simulink model "pendeLAI"  (Simulink 6.0)
settings: Solver=ode45  StartTime=0.0  StopTime=100.0  RelTol=1e-4
values from neighbouring files (symbols this model uses):
  PMswitch = 1    [quadresp_sim.m]    (also in quadresp_sim_2.m)
  UIMswitch = 1    [quadresp_sim.m]    (also in quadresp_sim_2.m)
libraries: cstblocks x15
settings Model: Creator=rana  LastModifiedBy=Administrator  ExtModeTrigMode=oneshot  ExtModeArmWhenConnect=off  ExtModeAutoUpdateStatusClock=off
settings DataIOCC: LimitDataPoints=off
settings OptimizationCC: BlockReduction=off  BooleanDataType=off
settings DebuggingCC: SolverPrmCheckMsg=none  UnconnectedInputMsg=none  UnconnectedOutputMsg=none
settings HardwareCC: TargetUnknown=on
settings GRTTargetCC: ModelReferenceCompliant=off  MatFileLogging=off

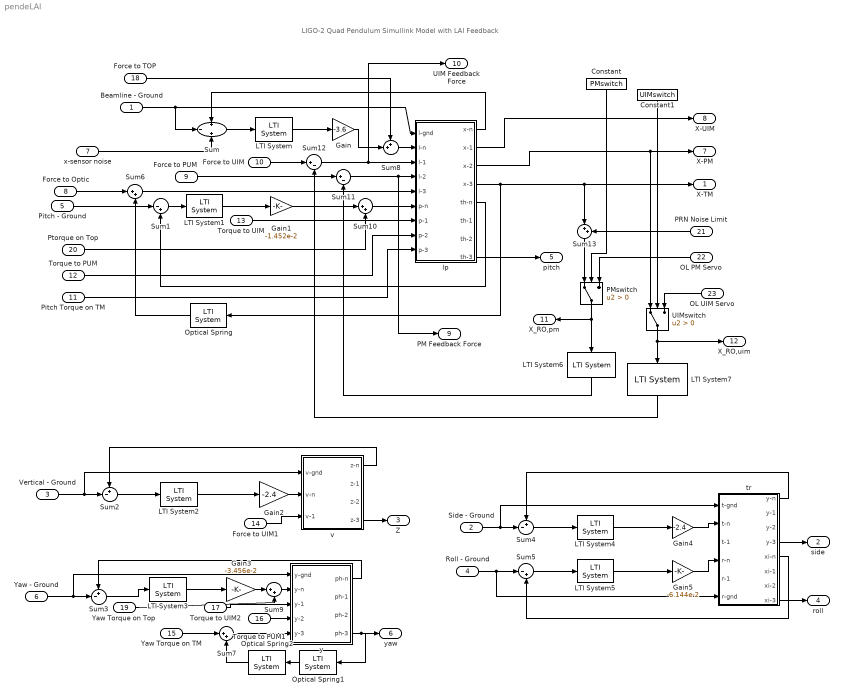
== system pendeLAI ==
  note: LIGO-2 Quad Pendulum Simullink Model
      | with LAI Feedback
  Beamline - Ground : Inport  Port=1  LatchInput=off
  Side - Ground : Inport  Port=2  LatchInput=off
  Vertical - Ground : Inport  Port=3  LatchInput=off
  Roll - Ground : Inport  Port=4  LatchInput=off
  Pitch - Ground : Inport  Port=5  LatchInput=off
  Yaw - Ground : Inport  Port=6  LatchInput=off
  x-sensor noise : Inport  Port=7  LatchInput=off
  Force to Optic : Inport  Port=8  LatchInput=off
  Force to PUM : Inport  Port=9  LatchInput=off
  Force to UIM : Inport  Port=10  LatchInput=off
  Pitch Torque on TM : Inport  Port=11  LatchInput=off
  Torque to PUM : Inport  Port=12  LatchInput=off
  Torque to UIM : Inport  Port=13  LatchInput=off
  Force to UIM1 : Inport  Port=14  LatchInput=off
  Yaw Torque on TM : Inport  Port=15  LatchInput=off
  Torque to PUM1 : Inport  Port=16  LatchInput=off
  Torque to UIM2 : Inport  Port=17  LatchInput=off
  Force to TOP : Inport  Port=18  LatchInput=off
  Yaw Torque on Top : Inport  Port=19  LatchInput=off
  Ptorque on Top : Inport  Port=20  LatchInput=off
  PRN Noise Limit : Inport  Orientation=left  Port=21  LatchInput=off
  OL PM Servo : Inport  Orientation=left  Port=22  LatchInput=off
  OL UIM Servo : Inport  Orientation=left  Port=23  LatchInput=off
  Constant : Constant  Orientation=down  Value=PMswitch
  Constant1 : Constant  Orientation=down  Value=UIMswitch
  Gain : Gain  Gain=-3.6
  Gain1 : Gain  Gain=-1.452e-2
  Gain2 : Gain  Gain=-2.4
  Gain3 : Gain  Gain=-3.456e-2
  Gain4 : Gain  Gain=-2.4
  Gain5 : Gain  Gain=-6.144e-2
  LTI System : cstblocks/LTI System  sys=ldamp  IC=0
  LTI System1 : cstblocks/LTI System  sys=pdamp  IC=0
  LTI System2 : cstblocks/LTI System  sys=vdamp  IC=0
  LTI System3 : cstblocks/LTI System  sys=ydamp  IC=0
  LTI System4 : cstblocks/LTI System  sys=tdamp  IC=0
  LTI System5 : cstblocks/LTI System  sys=rdamp  IC=0
  LTI System6 : cstblocks/LTI System  Orientation=down  sys=ServoPM  IC=[]
  LTI System7 : cstblocks/LTI System  Orientation=down  sys=ServoUIM  IC=[]
  Optical Spring : cstblocks/LTI System  Orientation=left  sys=k_ospring  IC=[]
  Optical Spring1 : cstblocks/LTI System  Orientation=left  sys=k_major  IC=[]
  Optical Spring2 : cstblocks/LTI System  Orientation=left  sys=k_minor  IC=[]
  PMswitch : Switch  Orientation=down  Criteria=u2 > Threshold
  Sum : Sum  Inputs=+|-|+  InputSameDT=on
  Sum1 : Sum  Inputs=|-+  InputSameDT=on
  Sum{6..7,9..10} (4 alike) : Sum  Inputs=|++  InputSameDT=on
  Sum11 : Sum  Inputs=|+-  InputSameDT=on
  Sum12 : Sum  Inputs=|+-  InputSameDT=on
  Sum13 : Sum  Orientation=down  Inputs=|++  InputSameDT=on
  Sum2 : Sum  Inputs=+-|  InputSameDT=on
  Sum3 : Sum  Inputs=+-|  InputSameDT=on
  Sum4 : Sum  Inputs=+-|  InputSameDT=on
  Sum5 : Sum  Inputs=|-+  InputSameDT=on
  Sum8 : Sum  Inputs=++|  InputSameDT=on
  UIMswitch : Switch  Orientation=down  Criteria=u2 > Threshold
  lp : Subsystem
  tr : Subsystem
  v : Subsystem
  y : Subsystem
  X-TM : Outport
  side : Outport  Port=2
  Z : Outport  Port=3
  roll : Outport  Port=4
  pitch : Outport  Port=5
  yaw : Outport  Port=6
  X-PM : Outport  Port=7
  X-UIM : Outport  Port=8
  PM Feedback Force : Outport  Port=9
  UIM Feedback Force : Outport  Port=10
  X_RO,pm : Outport  Orientation=left  Port=11
  X_RO,uim : Outport  Port=12
  wires:
  Gain2/1 -> v/2(v-n)
  Gain4/1 -> tr/2(t-n)
  Gain5/1 -> tr/4(r-n)
  Gain1/1 -> Sum10/1
  y/1(ph-n) -> Sum3/1
  tr/5(xi-n) -> Sum5/2
  tr/1(y-n) -> Sum4/1
  lp/5(th-n) -> Sum1/2
  lp/1(x-n) -> Sum/1
  LTI System/1 -> Gain/1
  Sum1/1 -> LTI System1/1
  Sum3/1 -> LTI System3/1
  Sum4/1 -> LTI System4/1
  Sum5/1 -> LTI System5/1
  v/1(z-n) -> Sum2/1
  Sum/1 -> LTI System/1
  Sum2/1 -> LTI System2/1
  Beamline - Ground/1 -> lp/1(l-gnd), Sum/2
  Pitch - Ground/1 -> Sum1/1
  Vertical - Ground/1 -> Sum2/2, v/1(v-gnd)
  Yaw - Ground/1 -> Sum3/2, y/1(y-gnd)
  Side - Ground/1 -> Sum4/2, tr/1(t-gnd)
  Roll - Ground/1 -> Sum5/1, tr/6(r-gnd)
  lp/4(x-3) -> Optical Spring/1, X-TM/1, Sum13/1
  tr/4(y-3) -> side/1
  v/4(z-3) -> Z/1
  tr/8(xi-3) -> roll/1
  lp/8(th-3) -> pitch/1
  y/4(ph-3) -> Optical Spring1/1, yaw/1
  LTI System1/1 -> Gain1/1
  LTI System2/1 -> Gain2/1
  LTI System3/1 -> Gain3/1
  LTI System4/1 -> Gain4/1
  LTI System5/1 -> Gain5/1
  x-sensor noise/1 -> Sum/3
  Pitch Torque on TM/1 -> lp/9(p-3)
  Torque to PUM/1 -> lp/8(p-2)
  Torque to UIM/1 -> lp/7(p-1)
  Force to Optic/1 -> Sum6/1
  Sum6/1 -> lp/5(l-3)
  Optical Spring/1 -> Sum6/2
  Force to UIM1/1 -> v/3(v-1)
  Torque to UIM2/1 -> y/3(y-1)
  Torque to PUM1/1 -> y/4(y-2)
  Yaw Torque on TM/1 -> Sum7/1
  Sum7/1 -> y/5(y-3)
  Optical Spring1/1 -> Optical Spring2/1
  Optical Spring2/1 -> Sum7/2
  Gain/1 -> Sum8/2
  Sum8/1 -> lp/2(I-n)
  Force to TOP/1 -> Sum8/1
  Gain3/1 -> Sum9/1
  Sum9/1 -> y/2(y-n)
  Yaw Torque on Top/1 -> Sum9/2
  Sum10/1 -> lp/6(p-n)
  Ptorque on Top/1 -> Sum10/2
  lp/3(x-2) -> X-PM/1, UIMswitch/1
  lp/2(x-1) -> X-UIM/1
  Sum11/1 -> lp/4(l-2), PM Feedback Force/1
  Force to PUM/1 -> Sum11/1
  LTI System6/1 -> Sum11/2
  Sum12/1 -> lp/3(l-1), UIM Feedback Force/1
  Force to UIM/1 -> Sum12/1
  LTI System7/1 -> Sum12/2
  PMswitch/1 -> LTI System6/1, X_RO,pm/1
  Sum13/1 -> PMswitch/1
  Constant/1 -> PMswitch/2
  OL PM Servo/1 -> PMswitch/3
  UIMswitch/1 -> LTI System7/1, X_RO,uim/1
  Constant1/1 -> UIMswitch/2
  OL UIM Servo/1 -> UIMswitch/3
  PRN Noise Limit/1 -> Sum13/2

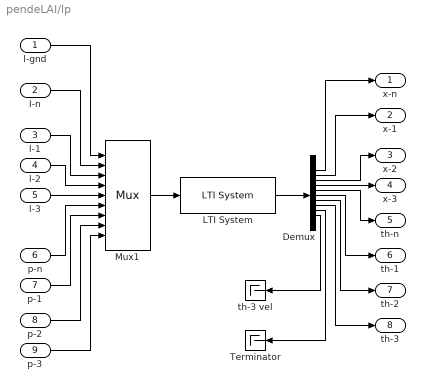
== system pendeLAI/lp ==
  l-gnd : Inport  Port=1  LatchInput=off
  I-n : Inport  Port=2  LatchInput=off
  l-1 : Inport  Port=3  LatchInput=off
  l-2 : Inport  Port=4  LatchInput=off
  l-3 : Inport  Port=5  LatchInput=off
  p-n : Inport  Port=6  LatchInput=off
  p-1 : Inport  Port=7  LatchInput=off
  p-2 : Inport  Port=8  LatchInput=off
  p-3 : Inport  Port=9  LatchInput=off
  Demux : Demux  Outputs=10
  LTI System : cstblocks/LTI System  sys=lpe  IC=[0]
  Mux1 : Mux  Inputs=9
      settings: DisplayOption=signals
  Terminator : Terminator
  th-3 vel : Terminator
  x-n : Outport
  x-1 : Outport  Port=2
  x-2 : Outport  Port=3
  x-3 : Outport  Port=4
  th-n : Outport  Port=5
  th-1 : Outport  Port=6
  th-2 : Outport  Port=7
  th-3 : Outport  Port=8
  wires:
  Mux1/1 -> LTI System/1
  LTI System/1 -> Demux/1
  Demux/1 -> x-n/1
  Demux/2 -> x-1/1
  Demux/3 -> x-2/1
  Demux/4 -> x-3/1
  Demux/5 -> th-n/1
  Demux/6 -> th-1/1
  Demux/7 -> th-2/1
  Demux/8 -> th-3/1
  l-gnd/1 -> Mux1/1
  I-n/1 -> Mux1/2
  l-1/1 -> Mux1/3
  l-2/1 -> Mux1/4
  l-3/1 -> Mux1/5
  p-n/1 -> Mux1/6
  p-1/1 -> Mux1/7
  p-2/1 -> Mux1/8
  p-3/1 -> Mux1/9
  Demux/9 -> Terminator/1
  Demux/10 -> th-3 vel/1

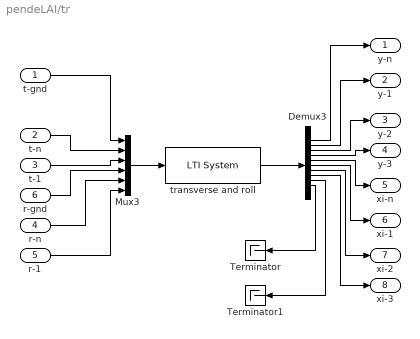
== system pendeLAI/tr ==
  t-gnd : Inport  Port=1  LatchInput=off
  t-n : Inport  Port=2  LatchInput=off
  t-1 : Inport  Port=3  LatchInput=off
  r-n : Inport  Port=4  LatchInput=off
  r-1 : Inport  Port=5  LatchInput=off
  r-gnd : Inport  Port=6  LatchInput=off
  Demux3 : Demux  Outputs=10
  Mux3 : Mux  Inputs=6
  Terminator : Terminator
  Terminator1 : Terminator
  transverse and roll : cstblocks/LTI System  sys=trer  IC=[0]
  y-n : Outport
  y-1 : Outport  Port=2
  y-2 : Outport  Port=3
  y-3 : Outport  Port=4
  xi-n : Outport  Port=5
  xi-1 : Outport  Port=6
  xi-2 : Outport  Port=7
  xi-3 : Outport  Port=8
  wires:
  Mux3/1 -> transverse and roll/1
  transverse and roll/1 -> Demux3/1
  Demux3/1 -> y-n/1
  Demux3/2 -> y-1/1
  Demux3/3 -> y-2/1
  Demux3/4 -> y-3/1
  Demux3/5 -> xi-n/1
  Demux3/6 -> xi-1/1
  Demux3/7 -> xi-2/1
  Demux3/8 -> xi-3/1
  t-gnd/1 -> Mux3/1
  t-n/1 -> Mux3/2
  t-1/1 -> Mux3/3
  r-1/1 -> Mux3/6
  r-n/1 -> Mux3/5
  r-gnd/1 -> Mux3/4
  Demux3/9 -> Terminator1/1
  Demux3/10 -> Terminator/1

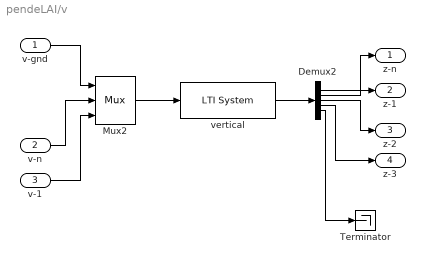
== system pendeLAI/v ==
  v-gnd : Inport  Port=1  LatchInput=off
  v-n : Inport  Port=2  LatchInput=off
  v-1 : Inport  Port=3  LatchInput=off
  Demux2 : Demux  Outputs=5
  Mux2 : Mux  Inputs=3
      settings: DisplayOption=signals
  Terminator : Terminator
  vertical : cstblocks/LTI System  sys=ve  IC=[0]
  z-n : Outport
  z-1 : Outport  Port=2
  z-2 : Outport  Port=3
  z-3 : Outport  Port=4
  wires:
  Mux2/1 -> vertical/1
  vertical/1 -> Demux2/1
  v-gnd/1 -> Mux2/1
  Demux2/1 -> z-n/1
  Demux2/2 -> z-1/1
  Demux2/3 -> z-2/1
  Demux2/4 -> z-3/1
  v-1/1 -> Mux2/3
  v-n/1 -> Mux2/2
  Demux2/5 -> Terminator/1

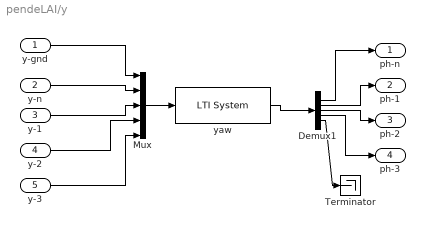
== system pendeLAI/y ==
  y-gnd : Inport  Port=1  LatchInput=off
  y-n : Inport  Port=2  LatchInput=off
  y-1 : Inport  Port=3  LatchInput=off
  y-2 : Inport  Port=4  LatchInput=off
  y-3 : Inport  Port=5  LatchInput=off
  Demux1 : Demux  Outputs=5
  Mux : Mux  Inputs=5
  Terminator : Terminator
  yaw : cstblocks/LTI System  sys=ye  IC=[0]
  ph-n : Outport
  ph-1 : Outport  Port=2
  ph-2 : Outport  Port=3
  ph-3 : Outport  Port=4
  wires:
  y-gnd/1 -> Mux/1
  Mux/1 -> yaw/1
  yaw/1 -> Demux1/1
  Demux1/1 -> ph-n/1
  Demux1/2 -> ph-1/1
  Demux1/3 -> ph-2/1
  Demux1/4 -> ph-3/1
  y-3/1 -> Mux/5
  y-2/1 -> Mux/4
  y-1/1 -> Mux/3
  y-n/1 -> Mux/2
  Demux1/5 -> Terminator/1
